simulink model "mophong_fuzzy"  (Simulink 8.0)
settings: Solver=ode3  StartTime=0.0  StopTime=100  FixedStep=0.01  RelTol=1e-2
values from neighbouring files (symbols this model uses):
  beta1 = 0.01122    [fuzzy_GA_25_9.m]
  beta2 = 0.00193    [fuzzy_GA_25_9.m]
  beta3 = 0.00156    [fuzzy_GA_25_9.m]
  beta4 = 0.0406    [fuzzy_GA_25_9.m]
  beta5 = 0.0078    [fuzzy_GA_25_9.m]
  g = 9.81    [fuzzy_GA_25_9.m]
  K1 = par(pop_index,1)    [fuzzy_GA_25_9.m]
  K2 = par(pop_index,2)    [fuzzy_GA_25_9.m]
  K3 = par(pop_index,3)    [fuzzy_GA_25_9.m]
  K4 = par(pop_index,4)    [fuzzy_GA_25_9.m]
  K5 = par(pop_index,5)    [fuzzy_GA_25_9.m]
  K6 = par(pop_index,6)    [fuzzy_GA_25_9.m]
  q1_dot_init = -0.02    [fuzzy_GA_25_9.m]
  q1_init = pi/2+0.01    (= 1.58079632679)    [fuzzy_GA_25_9.m]
  q2_dot_init = 0.024    [fuzzy_GA_25_9.m]
  q2_init = 0.01    [fuzzy_GA_25_9.m]
libraries: simulink x2, fuzblock x2
settings Model: Creator=KHACH  LastModifiedBy=user
settings SolverCC: ZeroCrossAlgorithm=Adaptive
settings DataIOCC: SignalLoggingSaveFormat=ModelDataLogs
settings DebuggingCC: FcnCallInpInsideContextMsg=UseLocalSettings  StrictBusMsg=Warning
settings GRTTargetCC: CombineOutputUpdateFcns=off  GRTInterface=on

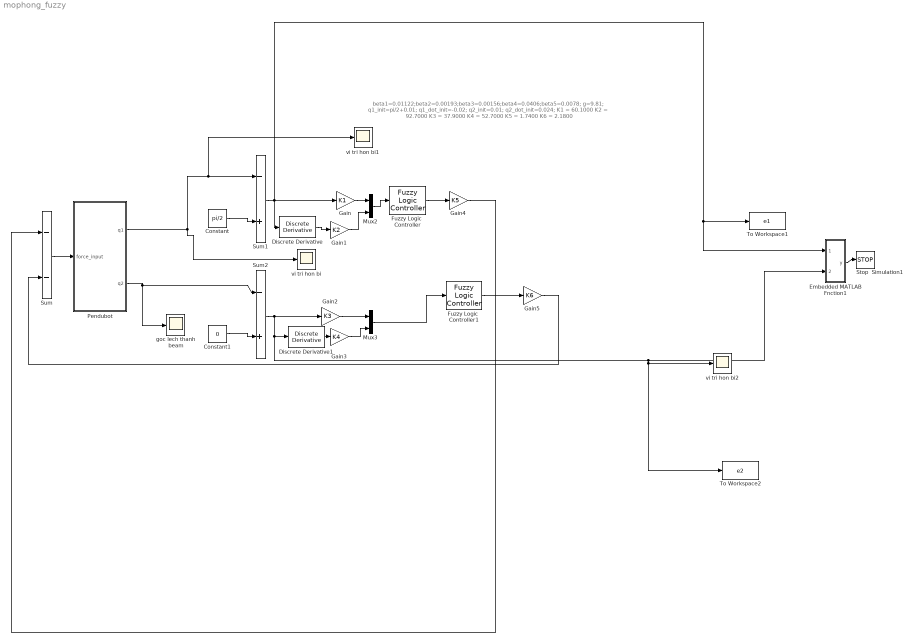
== system mophong_fuzzy ==
  note: beta1=0.01122;beta2=0.00193;beta3=0.00156;beta4=0.0406;beta5=0.0078;
      | g=9.81;
      | q1_init=pi/2+0.01;
      | q1_dot_init=-0.02;
      | q2_init=0.01;
      | q2_dot_init=0.024;
      | K1 =   60.1000
      | K2 =   92.7000
      | K3 =   37.9000
      | K4 =   52.7000
      | K5 =    1.7400
      | K6 =    2.1800
  Constant : Constant  Value=pi/2
  Constant1 : Constant  Value=0
  Discrete Derivative : simulink/Discrete/Discrete Derivative  gainval=1.0  ICPrevScaledInput=0.0  InputProcessing=Inherited  OutMin=[]  OutMax=[]  OutDataType=fixdt(1, 16)  OutScaling=2^-10  DoSatur=off
  Discrete Derivative1 : simulink/Discrete/Discrete Derivative  gainval=1.0  ICPrevScaledInput=0.0  InputProcessing=Inherited  OutMin=[]  OutMax=[]  OutDataType=fixdt(1, 16)  OutScaling=2^-10  DoSatur=off
  Embedded MATLAB Fnction1 : MATLAB Function  TreatAsAtomicUnit=on
  Fuzzy Logic  Controller : fuzblock/Fuzzy Logic  Controller  fis='mo_TueTam.fis'
  Fuzzy Logic  Controller1 : fuzblock/Fuzzy Logic  Controller  fis='mo_TueTam.fis'
  Gain : Gain  Gain=K1
  Gain1 : Gain  Gain=K2
  Gain2 : Gain  Gain=K3
  Gain3 : Gain  Gain=K4
  Gain4 : Gain  Gain=K5
  Gain5 : Gain  Gain=K6
  Mux2 : Mux  Inputs=2
  Mux3 : Mux  Inputs=2
  Pendubot : Subsystem
  Stop  Simulation1 : Stop
  Sum : Sum  Inputs=--
  Sum1 : Sum  Inputs=-+
  Sum2 : Sum  Inputs=-+
  To Workspace1 : ToWorkspace  VariableName=e1  SampleTime=-1
  To Workspace2 : ToWorkspace  VariableName=e2  SampleTime=-1
  goc lech thanh beam : Scope
      settings: SaveName=ScopeData5
  vi tri hon bi : Scope
      settings: TimeRange=40  YMin=-0.1  YMax=0.225  SaveName=ScopeData4
  vi tri hon bi1 : Scope
      settings: TimeRange=40  YMin=-0.1  YMax=0.225
  vi tri hon bi2 : Scope
      settings: TimeRange=40  YMin=-0.1  YMax=0.225
  wires:
  Sum/1 -> Pendubot/1(force_input)
  Fuzzy Logic  Controller/1 -> Gain4/1
  Pendubot/1(q1) -> vi tri hon bi/1, vi tri hon bi1/1, Sum1/1
  Pendubot/2(q2) -> Sum2/1, goc lech thanh beam/1
  Constant/1 -> Sum1/2
  Constant1/1 -> Sum2/2
  Fuzzy Logic  Controller1/1 -> Gain5/1
  Mux2/1 -> Fuzzy Logic  Controller/1
  Mux3/1 -> Fuzzy Logic  Controller1/1
  Discrete Derivative1/1 -> Gain3/1
  Gain/1 -> Mux2/1
  Discrete Derivative/1 -> Gain1/1
  Gain1/1 -> Mux2/2
  Gain2/1 -> Mux3/1
  Gain3/1 -> Mux3/2
  Gain4/1 -> Sum/1
  Gain5/1 -> Sum/2
  Embedded MATLAB Fnction1/1(y) -> Stop  Simulation1/1
  Sum2/1 -> Gain2/1, To Workspace2/1, vi tri hon bi2/1, Embedded MATLAB Fnction1/2(e2), Discrete Derivative1/1
  Sum1/1 -> To Workspace1/1, Embedded MATLAB Fnction1/1(e1), Discrete Derivative/1, Gain/1

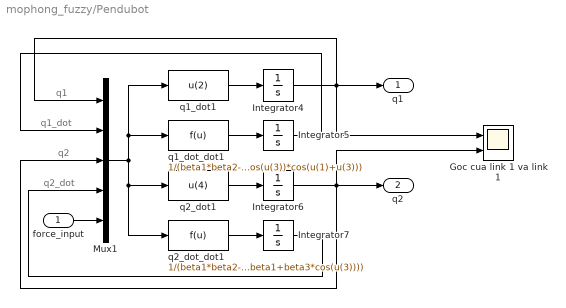
== system mophong_fuzzy/Pendubot ==
  note: q2_dot
  note: q2
  note: q1_dot
  note: q1
  force_input : Inport
  Goc cua link 1 va link 1 : Scope  NumInputPorts=2
      settings: YMin=-8200~12000  YMax=-6500~32000  SaveName=ScopeData2
  Integrator4 : Integrator  InitialCondition=q1_init  UpperSaturationLimit=pi  LowerSaturationLimit=-pi
  Integrator5 : Integrator  InitialCondition=q1_dot_init
  Integrator6 : Integrator  InitialCondition=q2_init  UpperSaturationLimit=pi  LowerSaturationLimit=-pi
  Integrator7 : Integrator  InitialCondition=q2_dot_init
  Mux1 : Mux  Inputs=5
  q1_dot1 : Fcn  Expr=u(2)
  q1_dot_dot1 : Fcn  Expr=1/(beta1*beta2-beta3^2*(cos(u(3)))^2)*(beta2*u(5)+beta2*beta3*sin(u(3))*(u(4)+u(2))^2+beta3^2*sin(u(3))*cos(u(3))*u(2)^2-beta2*beta4*g*cos(u(1))+beta3*beta5*g*cos(u(3))*cos(u(1)+u(3)))
  q2_dot1 : Fcn  Expr=u(4)
  q2_dot_dot1 : Fcn  Expr=1/(beta1*beta2-beta3^2*(cos(u(3)))^2)*(-beta2*u(5)-u(5)*beta3*cos(u(3))-beta3*sin(u(3))*(beta2+beta3*cos(u(3)))*(u(4)+u(2))^2-beta5*g*(beta1+beta3*cos(u(3)))*cos(u(1)+u(3))+beta4*g*(beta2+beta3*cos(u(3)))*cos(u(1))-beta3*(u(2))^2*sin(u(3))*(beta1+beta3*cos(u(3))))
  q1 : Outport
  q2 : Outport  Port=2
  wires:
  force_input/1 -> Mux1/5
  Mux1/1 -> q1_dot_dot1/1, q1_dot1/1, q2_dot_dot1/1, q2_dot1/1
  q1_dot_dot1/1 -> Integrator5/1
  Integrator6/1 -> Goc cua link 1 va link 1/2, Mux1/3, q2/1
  q2_dot_dot1/1 -> Integrator7/1
  Integrator4/1 -> Mux1/1, Goc cua link 1 va link 1/1, q1/1
  Integrator7/1 -> Mux1/4
  Integrator5/1 -> Mux1/2
  q2_dot1/1 -> Integrator6/1
  q1_dot1/1 -> Integrator4/1

== matlab function Embedded MATLAB Fnction1 ==
  data: e1 input double; y output double; e2 input double
function y = fcn(e1,e2)
if (abs(e1)>(100))||(abs(e2)>(100))
    y=1;
else
    y=0;
end
